simulink model "LQR_test_discrete"  (R2023b)
settings: Solver=ode4  StartTime=0.0  StopTime=10.0  RelTol=1e-3
values from neighbouring files (symbols this model uses):
  K = lqr(ss_continous.A, ss_continous.B, Q, R)    [LQR_tuning_continous.m]    (also in LQR_tuning_discrete.m = dlqr(ss_object_discrete.A, ss_object_discrete.B, Q, R))
  ss_object_discrete = c2d(ss(ss_continous.A, ss_continous.B, ss_continous.C, ss_continous.D), Ts, 'zoh')    [closed_loop_identification_P.m]    (also in closed_loop_identification_RK4.m)
  Ts = 0.001    [init.m]
undefined symbols (not defined in the file or in its folder): Discrete, Time
libraries: simulink x1, ctrlSharedLib x1
settings Model: Creator=User  LastModifiedBy=User

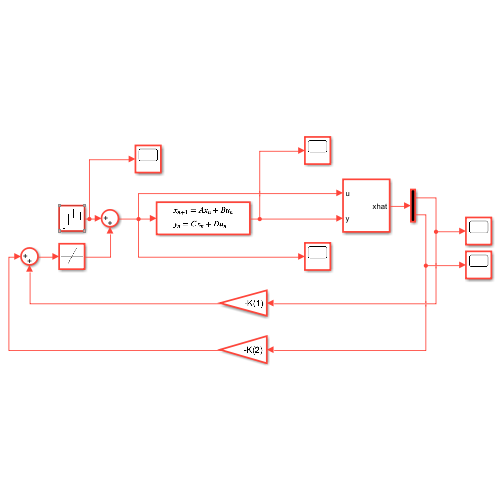
[thumbnail: Simulink's stored preview of the top-level diagram]
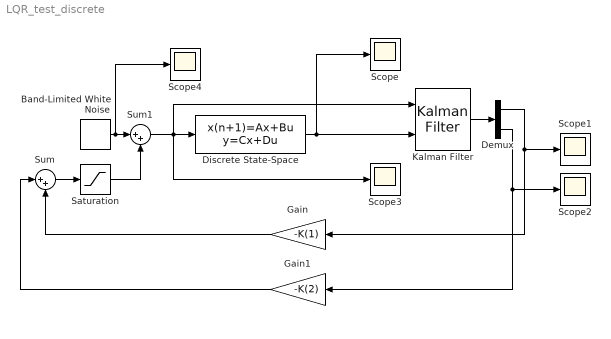
== system LQR_test_discrete ==
  Band-Limited White Noise : simulink/Sources/Band-Limited White Noise  Cov=[1.0]  Ts=Ts  seed=[23341]
  Demux : Demux  Outputs=2
  Discrete State-Space : DiscreteStateSpace  A=ss_object_discrete.A  B=ss_object_discrete.B  C=ss_object_discrete.C  D=ss_object_discrete.D  SampleTime=-1
  Gain : Gain  Gain=-K(1)
  Gain1 : Gain  Gain=-K(2)
  Kalman Filter : ctrlSharedLib/Kalman Filter  TimeDomain=Discrete-Time  UseCurrentEstimator=on  ModelSource=Individual A, B, C, D matrices  ModelSourceVariable=ss(0.95,1,1,0,1)  A=ss_object_discrete.A  B=ss_object_discrete.B  C=ss_object_discrete.C  D=ss_object_discrete.D  NumberOfStates=1  NumberOfInputs=1  NumberOfOutputs=1  InitialEstimateSource=Dialog  X0=0  P0=10  UseK=off  UseGH=off  NumberOfProcessNoiseInputs=1  G=1  TimeInvariantG=on  H=0  TimeInvariantH=on  Q=0.05  TimeInvariantQ=on  R=1  TimeInvariantR=on  N=0  TimeInvariantN=on  AddInputPort=on  AddEnablePort=off  OutputEstimatedY=off  OutputP=off  Ts=-1
  Saturation : Saturate  UpperLimit=100  LowerLimit=-100
  Scope{,1..4} (5 alike) : Scope
  Sum : Sum  Inputs=|++
  Sum1 : Sum  Inputs=|++
  wires:
  Discrete State-Space/1 -> Scope/1, Kalman Filter/2
  Gain/1 -> Sum/2
  Gain1/1 -> Sum/1
  Sum1/1 -> Kalman Filter/1, Scope3/1, Discrete State-Space/1
  Kalman Filter/1 -> Demux/1
  Demux/1 -> Scope1/1, Gain/1
  Demux/2 -> Scope2/1, Gain1/1
  Saturation/1 -> Sum1/2
  Sum/1 -> Saturation/1
  Band-Limited White Noise/1 -> Scope4/1, Sum1/1
